simulink library "adrc_lib"  (R2017a)
settings: Solver=VariableStepAuto  StartTime=0.0  StopTime=10.0  RelTol=1e-3
undefined symbols (not defined in the file): alpha, delta, DiscIntNeverNeededParam, h, h0, J, K, r0
libraries: simulink_extras x2, adrc_lib x1
settings Model: Creator=uids8840  LastModifiedBy=root

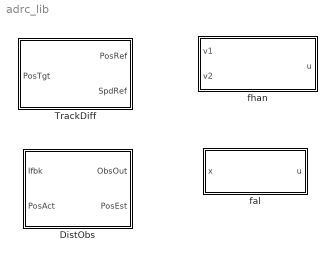
== system adrc_lib ==
  DistObs : Subsystem  SystemSampleTime=1/30e3  mask{k0=-800, k1=-25, k2=-1/4, Jest=J, Kest=K, ts=1/30e3}
      mask prompts: Jest "Motor Inertia [J]"; Kest "Motor Constant [K]"; ts "Execution rate [s]"
  TrackDiff : Subsystem  mask{ts=1e-3, r0=1e3}
      mask prompts: ts "Exeuction rate [s]:"; r0 "Agressivenes [r0]"
      mask init:
      | h0 = ts;
  fal : Subsystem
  fhan : Subsystem

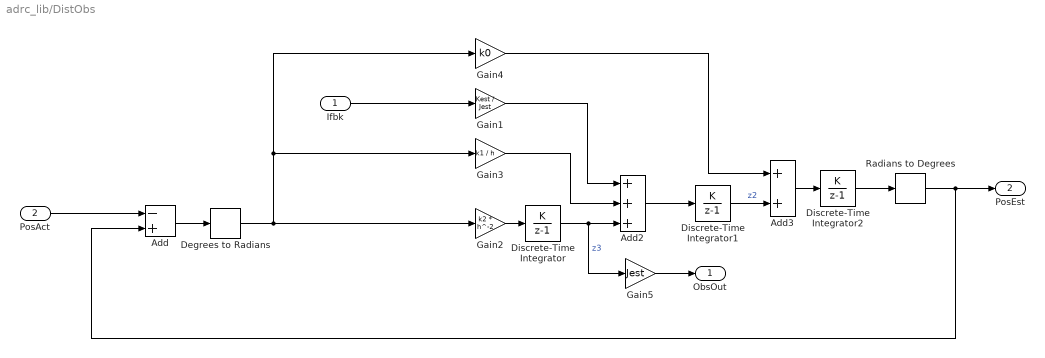
== system adrc_lib/DistObs ==
  Ifbk : Inport
  PosAct : Inport  Port=2
  Add : Sum  Inputs=-+
  Add2 : Sum  Inputs=+++
  Add3 : Sum
  Degrees to Radians : simulink_extras/Transformations/Degrees to Radians
  Discrete-Time Integrator : DiscreteIntegrator  IntegratorMethod=Accumulation: Forward Euler  gainval=ts  SampleTime=-1  ICPrevOutput=DiscIntNeverNeededParam  ICPrevScaledInput=DiscIntNeverNeededParam
  Discrete-Time Integrator1 : DiscreteIntegrator  IntegratorMethod=Accumulation: Forward Euler  gainval=ts  SampleTime=-1  ICPrevOutput=DiscIntNeverNeededParam  ICPrevScaledInput=DiscIntNeverNeededParam
  Discrete-Time Integrator2 : DiscreteIntegrator  IntegratorMethod=Accumulation: Forward Euler  gainval=ts  SampleTime=-1  ICPrevOutput=DiscIntNeverNeededParam  ICPrevScaledInput=DiscIntNeverNeededParam
  Gain1 : Gain  Gain=Kest / Jest
  Gain2 : Gain  Gain=k2 * h^-2
  Gain3 : Gain  Gain=k1 / h
  Gain4 : Gain  Gain=k0
  Gain5 : Gain  Gain=Jest
  Radians to Degrees : simulink_extras/Transformations/Radians to Degrees
  ObsOut : Outport
  PosEst : Outport  Port=2
  wires:
  Ifbk/1 -> Gain1/1
  Gain2/1 -> Discrete-Time Integrator/1
  Gain1/1 -> Add2/1
  Add2/1 -> Discrete-Time Integrator1/1
  Gain4/1 -> Add3/1
  Discrete-Time Integrator/1 -> Add2/3, Gain5/1  "z3"
  Add3/1 -> Discrete-Time Integrator2/1
  Gain3/1 -> Add2/2
  Discrete-Time Integrator1/1 -> Add3/2  "z2"
  Add/1 -> Degrees to Radians/1
  PosAct/1 -> Add/1
  Discrete-Time Integrator2/1 -> Radians to Degrees/1
  Radians to Degrees/1 -> Add/2, PosEst/1
  Degrees to Radians/1 -> Gain2/1, Gain4/1, Gain3/1
  Gain5/1 -> ObsOut/1

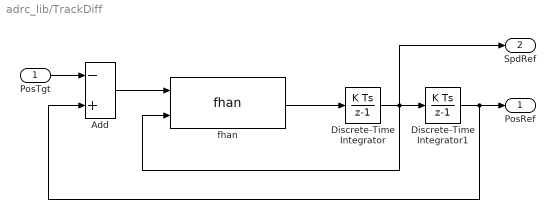
== system adrc_lib/TrackDiff ==
  PosTgt : Inport
  Add : Sum  Inputs=-+
  Discrete-Time Integrator : DiscreteIntegrator  InitialConditionSetting=State (most efficient)  SampleTime=ts  ICPrevOutput=DiscIntNeverNeededParam  ICPrevScaledInput=DiscIntNeverNeededParam
  Discrete-Time Integrator1 : DiscreteIntegrator  InitialConditionSetting=State (most efficient)  SampleTime=ts  ICPrevOutput=DiscIntNeverNeededParam  ICPrevScaledInput=DiscIntNeverNeededParam
  fhan : adrc_lib/fhan
  PosRef : Outport
  SpdRef : Outport  Port=2
  wires:
  Discrete-Time Integrator1/1 -> PosRef/1, Add/2
  Discrete-Time Integrator/1 -> fhan/2, Discrete-Time Integrator1/1, SpdRef/1
  fhan/1 -> Discrete-Time Integrator/1
  Add/1 -> fhan/1
  PosTgt/1 -> Add/1

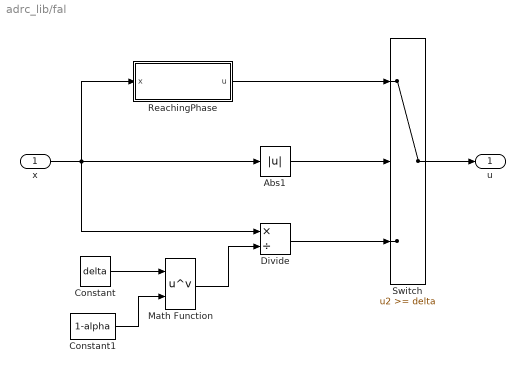
== system adrc_lib/fal ==
  x : Inport
  Abs1 : Abs
  Constant : Constant  Value=delta
  Constant1 : Constant  Value=1-alpha
  Divide : Product  Inputs=*/
  Math Function : Math  Operator=pow  SaturateOnIntegerOverflow=on
  ReachingPhase : Subsystem
  Switch : Switch  Threshold=delta
      settings: AttributesFormatString=%<Criteria>
  u : Outport
  wires:
  x/1 -> ReachingPhase/1(x), Divide/1, Abs1/1
  Divide/1 -> Switch/3
  Constant/1 -> Math Function/1
  Math Function/1 -> Divide/2
  Switch/1 -> u/1
  Abs1/1 -> Switch/2
  Constant1/1 -> Math Function/2
  ReachingPhase/1(u) -> Switch/1

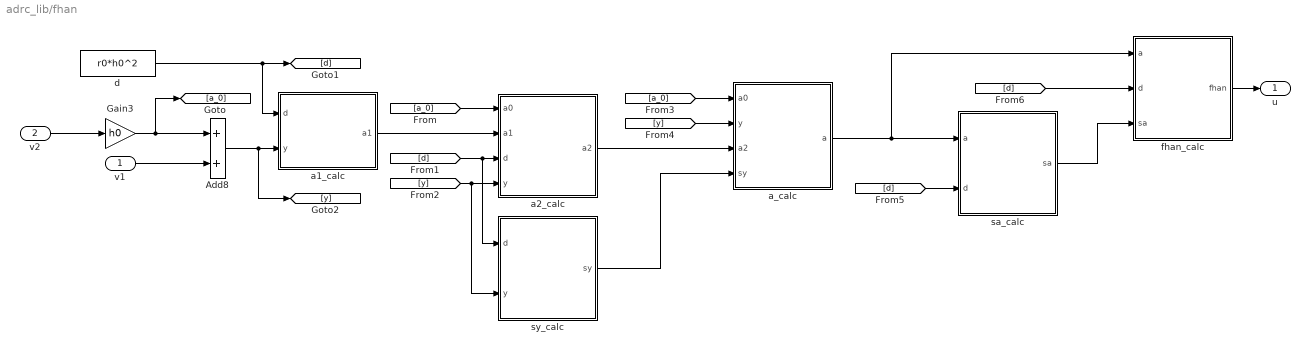
== system adrc_lib/fhan ==
  v1 : Inport
  v2 : Inport  Port=2
  Add8 : Sum
  Gain3 : Gain  Gain=h0
  a1_calc : Subsystem
  a2_calc : Subsystem
  a_calc : Subsystem
  d : Constant  Value=r0*h0^2
  fhan_calc : Subsystem
  sa_calc : Subsystem
  sy_calc : Subsystem
  u : Outport
  wires:
  v1/1 -> Add8/2
  v2/1 -> Gain3/1
  sy_calc/1(sy) -> a_calc/4(sy)
  [d] -> sa_calc/2(d)
  [d] -> a2_calc/3(d), sy_calc/1(d)
  [y] -> a2_calc/4(y), sy_calc/2(y)
  sa_calc/1(sa) -> fhan_calc/3(sa)
  [d] -> fhan_calc/2(d)
  d/1 -> [d], a1_calc/1(d)
  Add8/1 -> a1_calc/2(y), [y]
  Gain3/1 -> [a_0], Add8/1
  fhan_calc/1(fhan) -> u/1
  a_calc/1(a) -> sa_calc/1(a), fhan_calc/1(a)
  [y] -> a_calc/2(y)
  a1_calc/1(a1) -> a2_calc/2(a1)
  [a_0] -> a2_calc/1(a0)
  [a_0] -> a_calc/1(a0)
  a2_calc/1(a2) -> a_calc/3(a2)

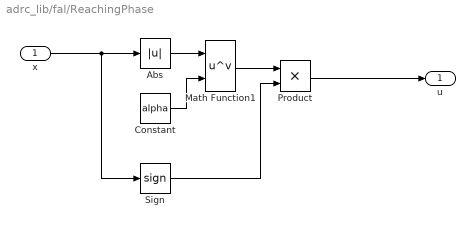
== system adrc_lib/fal/ReachingPhase ==
  x : Inport
  Abs : Abs
  Constant : Constant  Value=alpha
  Math Function1 : Math  Operator=pow  SaturateOnIntegerOverflow=on
  Product : Product
  Sign : Signum
  u : Outport
  wires:
  Product/1 -> u/1
  Math Function1/1 -> Product/1
  Abs/1 -> Math Function1/1
  Sign/1 -> Product/2
  Constant/1 -> Math Function1/2
  x/1 -> Sign/1, Abs/1

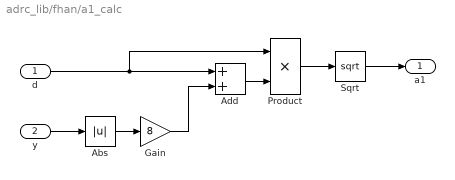
== system adrc_lib/fhan/a1_calc ==
  d : Inport
  y : Inport  Port=2
  Abs : Abs
  Add : Sum
  Gain : Gain  Gain=8
  Product : Product
  Sqrt : Sqrt  SaturateOnIntegerOverflow=on
  a1 : Outport
  wires:
  Sqrt/1 -> a1/1
  Product/1 -> Sqrt/1
  Add/1 -> Product/2
  Gain/1 -> Add/2
  Abs/1 -> Gain/1
  y/1 -> Abs/1
  d/1 -> Add/1, Product/1

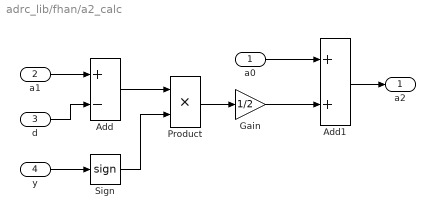
== system adrc_lib/fhan/a2_calc ==
  a0 : Inport
  a1 : Inport  Port=2
  d : Inport  Port=3
  y : Inport  Port=4
  Add : Sum  Inputs=+-
  Add1 : Sum
  Gain : Gain  Gain=1/2
  Product : Product
  Sign : Signum
  a2 : Outport
  wires:
  a0/1 -> Add1/1
  Gain/1 -> Add1/2
  Product/1 -> Gain/1
  Sign/1 -> Product/2
  Add/1 -> Product/1
  y/1 -> Sign/1
  d/1 -> Add/2
  a1/1 -> Add/1
  Add1/1 -> a2/1

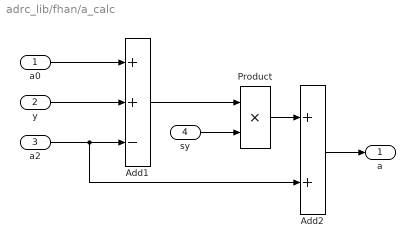
== system adrc_lib/fhan/a_calc ==
  a0 : Inport
  y : Inport  Port=2
  a2 : Inport  Port=3
  sy : Inport  Port=4
  Add1 : Sum  Inputs=++-
  Add2 : Sum
  Product : Product
  a : Outport
  wires:
  Product/1 -> Add2/1
  sy/1 -> Product/2
  Add1/1 -> Product/1
  a2/1 -> Add1/3, Add2/2
  y/1 -> Add1/2
  a0/1 -> Add1/1
  Add2/1 -> a/1

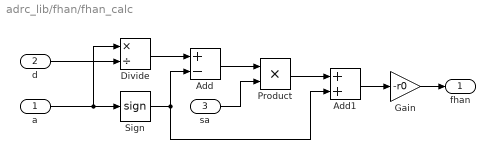
== system adrc_lib/fhan/fhan_calc ==
  a : Inport
  d : Inport  Port=2
  sa : Inport  Port=3
  Add : Sum  Inputs=+-
  Add1 : Sum
  Divide : Product  Inputs=*/
  Gain : Gain  Gain=-r0
  Product : Product
  Sign : Signum
  fhan : Outport
  wires:
  Product/1 -> Add1/1
  Add1/1 -> Gain/1
  sa/1 -> Product/2
  Add/1 -> Product/1
  Sign/1 -> Add/2, Add1/2
  Divide/1 -> Add/1
  a/1 -> Sign/1, Divide/1
  Gain/1 -> fhan/1
  d/1 -> Divide/2

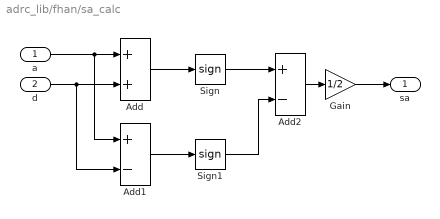
== system adrc_lib/fhan/sa_calc ==
  a : Inport
  d : Inport  Port=2
  Add : Sum
  Add1 : Sum  Inputs=+-
  Add2 : Sum  Inputs=+-
  Gain : Gain  Gain=1/2
  Sign : Signum
  Sign1 : Signum
  sa : Outport
  wires:
  Add2/1 -> Gain/1
  Sign1/1 -> Add2/2
  Sign/1 -> Add2/1
  Add1/1 -> Sign1/1
  Add/1 -> Sign/1
  a/1 -> Add/1, Add1/1
  d/1 -> Add1/2, Add/2
  Gain/1 -> sa/1

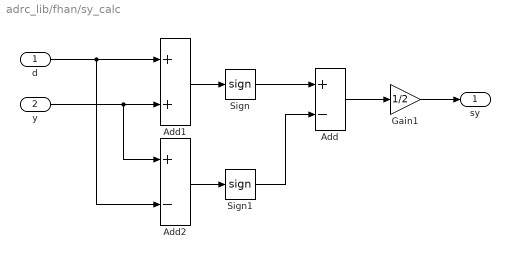
== system adrc_lib/fhan/sy_calc ==
  d : Inport
  y : Inport  Port=2
  Add : Sum  Inputs=+-
  Add1 : Sum
  Add2 : Sum  Inputs=+-
  Gain1 : Gain  Gain=1/2
  Sign : Signum
  Sign1 : Signum
  sy : Outport
  wires:
  Add/1 -> Gain1/1
  Add2/1 -> Sign1/1
  Sign1/1 -> Add/2
  Sign/1 -> Add/1
  Add1/1 -> Sign/1
  Gain1/1 -> sy/1
  d/1 -> Add1/1, Add2/2
  y/1 -> Add1/2, Add2/1
